simulink model "Proiect"  (R2023b)
settings: Solver=ode45  StartTime=0.0  StopTime=3600  RelTol=1e-3
values from neighbouring files (symbols this model uses):
  A = 332.5    [Proiect.m]
  C = 5.75    [Proiect.m]
  h = 12.99    [Proiect.m]
  h0 = 10.22    [Proiect.m]
  k = 0.025    [Proiect.m]
  k1 = 0.654    [Proiect.m]
  k11 = k2^2 + 4 * (k - k3) * k1    (= 0.0671946)    [Proiect.m]
  k12 = 8 * (k - k3)    (= 0.2048)    [Proiect.m]
  k13 = 2 * (k - k3)    (= 0.0512)    [Proiect.m]
  k2 = -0.015    [Proiect.m]
  k3 = -0.0006    [Proiect.m]
  k_compensare = kpFF/kp_comp    (= 0.13698630137)    [Proiect.m]
  k_eta = 8 * 10^(-5)    (= 8e-05)    [Proiect.m]
  ki2 = 0.184    [Proiect.m]
  kr = 2.1661    [Proiect.m]
  kr1 = Tf1/(kf1*T01)    (= 0.30303030303)    [Proiect.m]
  kr2 = Tf2/(kf2*T02)    (= 47.4368231047)    [Proiect.m]
  kre2 = 47.4    [Proiect.m]
  kri2 = 0.303    [Proiect.m]
  q = 32.45    [Proiect.m]
  q0 = 28.8    [Proiect.m]
  Ti = kr * 1/0.01589    (= 136.31843927)    [Proiect.m]
  Tr1 = Tf1    (= 0.76)    [Proiect.m]
  Tr2 = Tf2    (= 258.25)    [Proiect.m]
  u0 = 4.5    [Proiect.m]
libraries: slpidlib x12
(part 2 of 2)

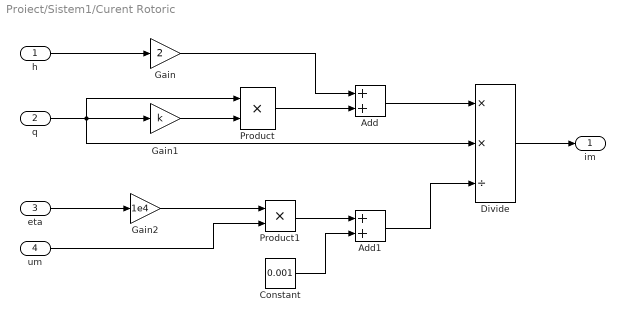
== system Proiect/Sistem1/Curent Rotoric ==
  h : Inport
  q : Inport  Port=2
  eta : Inport  Port=3
  um : Inport  Port=4
  Add : Sum
  Add1 : Sum
  Constant : Constant  Value=0.001
  Divide : Product  Inputs=**/
  Gain : Gain  Gain=2
  Gain1 : Gain  Gain=k
  Gain2 : Gain  Gain=1e4
  Product : Product
  Product1 : Product
  im : Outport
  wires:
  Gain1/1 -> Product/2
  Product/1 -> Add/2
  Gain2/1 -> Product1/1
  h/1 -> Gain/1
  Constant/1 -> Add1/2
  Gain/1 -> Add/1
  um/1 -> Product1/2
  Add1/1 -> Divide/3
  Divide/1 -> im/1
  Add/1 -> Divide/1
  q/1 -> Divide/2, Product/1, Gain1/1
  eta/1 -> Gain2/1
  Product1/1 -> Add1/1

== system Proiect/Sistem1/Filtru ==
  q : Inport
  Integrator : Integrator  InitialCondition=q0
  Sum : Sum  Inputs=|+-
  q_f : Outport
  wires:
  q/1 -> Sum/1
  Integrator/1 -> q_f/1, Sum/2
  Sum/1 -> Integrator/1

== system Proiect/Sistem1/Motor ==
  um : Inport
  im : Inport  Port=2
  Add : Sum  Inputs=+-
  Gain : Gain  Gain=3
  kn : Outport
  wires:
  im/1 -> Gain/1
  um/1 -> Add/1
  Add/1 -> kn/1
  Gain/1 -> Add/2

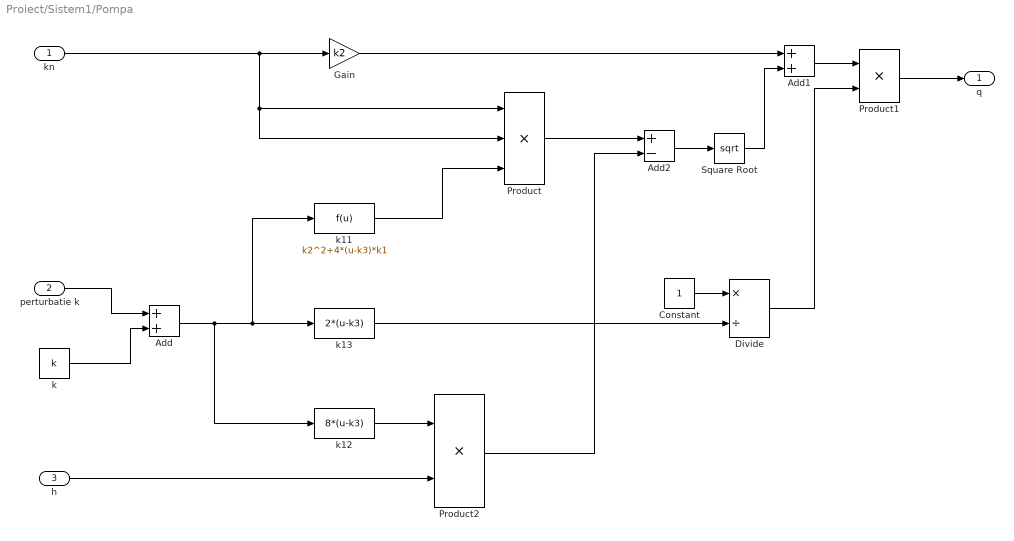
== system Proiect/Sistem1/Pompa ==
  kn : Inport
  perturbatie k : Inport  Port=2
  h : Inport  Port=3
  Add : Sum
  Add1 : Sum
  Add2 : Sum  Inputs=+-
  Constant : Constant
  Divide : Product  Inputs=*/
  Gain : Gain  Gain=k2
  Product : Product  Inputs=3
  Product1 : Product
  Product2 : Product
  Square Root : Sqrt
  k : Constant  Value=k
  k11 : Fcn  Expr=k2^2+4*(u-k3)*k1
  k12 : Fcn  Expr=8*(u-k3)
  k13 : Fcn  Expr=2*(u-k3)
  q : Outport
  wires:
  perturbatie k/1 -> Add/1
  k/1 -> Add/2
  k11/1 -> Product/3
  kn/1 -> Product/1, Product/2, Gain/1
  Gain/1 -> Add1/1
  Product/1 -> Add2/1
  Add2/1 -> Square Root/1
  Square Root/1 -> Add1/2
  Product1/1 -> q/1
  Add1/1 -> Product1/1
  Add/1 -> k12/1, k13/1, k11/1
  h/1 -> Product2/2
  Product2/1 -> Add2/2
  Constant/1 -> Divide/1
  k13/1 -> Divide/2
  Divide/1 -> Product1/2
  k12/1 -> Product2/1

== system Proiect/Sistem1/Randament Pompa ==
  q : Inport
  um : Inport  Port=2
  Gain : Gain  Gain=k_eta
  Product : Product
  eta : Outport
  wires:
  um/1 -> Gain/1
  Gain/1 -> Product/2
  Product/1 -> eta/1
  q/1 -> Product/1

== system Proiect/Sistem1/Rezervor ==
  q : Inport
  Fcn : Fcn  Expr=sqrt(u)*9
  Gain : Gain  Gain=1/A
  Integrator : Integrator  InitialCondition=h0
  Sum : Sum  Inputs=|+-
  h : Outport
  wires:
  Sum/1 -> Gain/1
  Integrator/1 -> Fcn/1, h/1
  q/1 -> Sum/1
  Gain/1 -> Integrator/1
  Fcn/1 -> Sum/2

== system Proiect/Sistem2/Amplificator ==
  ua : Inport
  Constant : Constant  Value=8.1
  Gain : Gain  Gain=2.2
  Gain1 : Gain  Gain=2.2
  Gain2 : Gain  Gain=5
  Saturation : Saturate  UpperLimit=22  LowerLimit=0
  Sum : Sum  Inputs=|++
  Sum1 : Sum  Inputs=|+-
  Switch : Switch  Threshold=8.1  SaturateOnIntegerOverflow=off  InputSameDT=off
  um : Outport
  wires:
  Switch/1 -> Saturation/1
  ua/1 -> Switch/2, Gain/1, Sum1/1, Gain1/1
  Gain1/1 -> Sum/1
  Gain2/1 -> Sum/2
  Saturation/1 -> um/1
  Gain/1 -> Switch/3
  Constant/1 -> Sum1/2
  Sum1/1 -> Gain2/1
  Sum/1 -> Switch/1

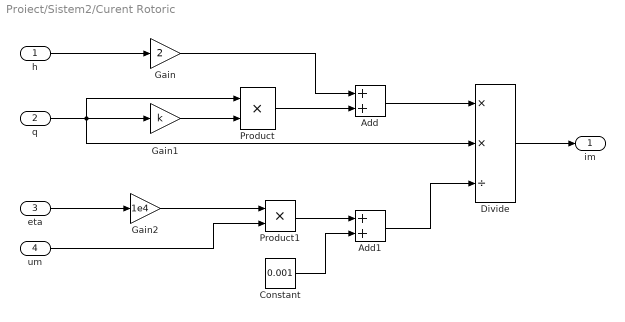
== system Proiect/Sistem2/Curent Rotoric ==
  h : Inport
  q : Inport  Port=2
  eta : Inport  Port=3
  um : Inport  Port=4
  Add : Sum
  Add1 : Sum
  Constant : Constant  Value=0.001
  Divide : Product  Inputs=**/
  Gain : Gain  Gain=2
  Gain1 : Gain  Gain=k
  Gain2 : Gain  Gain=1e4
  Product : Product
  Product1 : Product
  im : Outport
  wires:
  Gain1/1 -> Product/2
  Product/1 -> Add/2
  Gain2/1 -> Product1/1
  h/1 -> Gain/1
  Constant/1 -> Add1/2
  Gain/1 -> Add/1
  um/1 -> Product1/2
  Add1/1 -> Divide/3
  Divide/1 -> im/1
  Add/1 -> Divide/1
  q/1 -> Divide/2, Product/1, Gain1/1
  eta/1 -> Gain2/1
  Product1/1 -> Add1/1

== system Proiect/Sistem2/Filtru ==
  q : Inport
  Integrator : Integrator  InitialCondition=q0
  Sum : Sum  Inputs=|+-
  q_f : Outport
  wires:
  q/1 -> Sum/1
  Integrator/1 -> q_f/1, Sum/2
  Sum/1 -> Integrator/1

== system Proiect/Sistem2/Motor ==
  um : Inport
  im : Inport  Port=2
  Add : Sum  Inputs=+-
  Gain : Gain  Gain=3
  kn : Outport
  wires:
  im/1 -> Gain/1
  um/1 -> Add/1
  Add/1 -> kn/1
  Gain/1 -> Add/2

== system Proiect/Sistem2/Pompa ==
  kn : Inport
  h : Inport  Port=2
  Add : Sum
  Gain : Gain  Gain=k11
  Gain1 : Gain  Gain=k2
  Gain2 : Gain  Gain=1/k13
  Gain3 : Gain  Gain=k12
  Product : Product
  Square Root : Sqrt
  Subtract : Sum  Inputs=+-
  qi : Outport
  wires:
  Gain/1 -> Subtract/1
  Square Root/1 -> Add/2
  Gain3/1 -> Subtract/2
  Product/1 -> Gain/1
  Subtract/1 -> Square Root/1
  Gain2/1 -> qi/1
  kn/1 -> Product/1, Gain1/1, Product/2
  Add/1 -> Gain2/1
  Gain1/1 -> Add/1
  h/1 -> Gain3/1

== system Proiect/Sistem2/Randament Pompa ==
  q : Inport
  um : Inport  Port=2
  Gain : Gain  Gain=k_eta
  Product : Product
  eta : Outport
  wires:
  um/1 -> Gain/1
  Gain/1 -> Product/2
  Product/1 -> eta/1
  q/1 -> Product/1

== system Proiect/Sistem2/Rezervor ==
  q : Inport
  Add : Sum
  Constant : Constant  Value=C
  Gain : Gain  Gain=1/A
  Integrator : Integrator  InitialCondition=h0
  Product : Product
  Product1 : Product
  Square Root : Sqrt
  Step : Step  Time=500  After=2  SampleTime=0
  Sum : Sum  Inputs=|+-
  h : Outport
  perturbatie : Outport  Port=2
  qe : Outport  Port=3
  wires:
  Sum/1 -> Gain/1
  Integrator/1 -> Square Root/1, h/1
  q/1 -> Sum/1
  Gain/1 -> Integrator/1
  Product/1 -> qe/1, Sum/2
  Square Root/1 -> Product1/1, Product/1
  Add/1 -> Product/2
  Constant/1 -> Add/2
  Step/1 -> Product1/2, Add/1
  Product1/1 -> perturbatie/1

== system Proiect/Sistem3/Amplificator ==
  ua : Inport
  Constant : Constant  Value=8.1
  Gain : Gain  Gain=2.2
  Gain1 : Gain  Gain=2.2
  Gain2 : Gain  Gain=5
  Saturation : Saturate  UpperLimit=22  LowerLimit=0
  Sum : Sum  Inputs=|++
  Sum1 : Sum  Inputs=|+-
  Switch : Switch  Threshold=8.1  SaturateOnIntegerOverflow=off  InputSameDT=off
  um : Outport
  wires:
  Switch/1 -> Saturation/1
  ua/1 -> Switch/2, Gain/1, Sum1/1, Gain1/1
  Gain1/1 -> Sum/1
  Gain2/1 -> Sum/2
  Saturation/1 -> um/1
  Gain/1 -> Switch/3
  Constant/1 -> Sum1/2
  Sum1/1 -> Gain2/1
  Sum/1 -> Switch/1

== system Proiect/Sistem3/Curent Rotoric ==
  h : Inport
  q : Inport  Port=2
  eta : Inport  Port=3
  um : Inport  Port=4
  Add : Sum
  Add1 : Sum
  Constant : Constant  Value=0.001
  Divide : Product  Inputs=**/
  Gain : Gain  Gain=2
  Gain1 : Gain  Gain=k
  Gain2 : Gain  Gain=1e4
  Product : Product
  Product1 : Product
  im : Outport
  wires:
  Gain1/1 -> Product/2
  Product/1 -> Add/2
  Gain2/1 -> Product1/1
  h/1 -> Gain/1
  Constant/1 -> Add1/2
  Gain/1 -> Add/1
  um/1 -> Product1/2
  Add1/1 -> Divide/3
  Divide/1 -> im/1
  Add/1 -> Divide/1
  q/1 -> Divide/2, Product/1, Gain1/1
  eta/1 -> Gain2/1
  Product1/1 -> Add1/1

== system Proiect/Sistem3/Filtru ==
  q : Inport
  Integrator : Integrator  InitialCondition=q0
  Sum : Sum  Inputs=|+-
  q_f : Outport
  wires:
  q/1 -> Sum/1
  Integrator/1 -> q_f/1, Sum/2
  Sum/1 -> Integrator/1

== system Proiect/Sistem3/Motor ==
  um : Inport
  im : Inport  Port=2
  Add : Sum  Inputs=+-
  Gain : Gain  Gain=3
  kn : Outport
  wires:
  im/1 -> Gain/1
  um/1 -> Add/1
  Add/1 -> kn/1
  Gain/1 -> Add/2

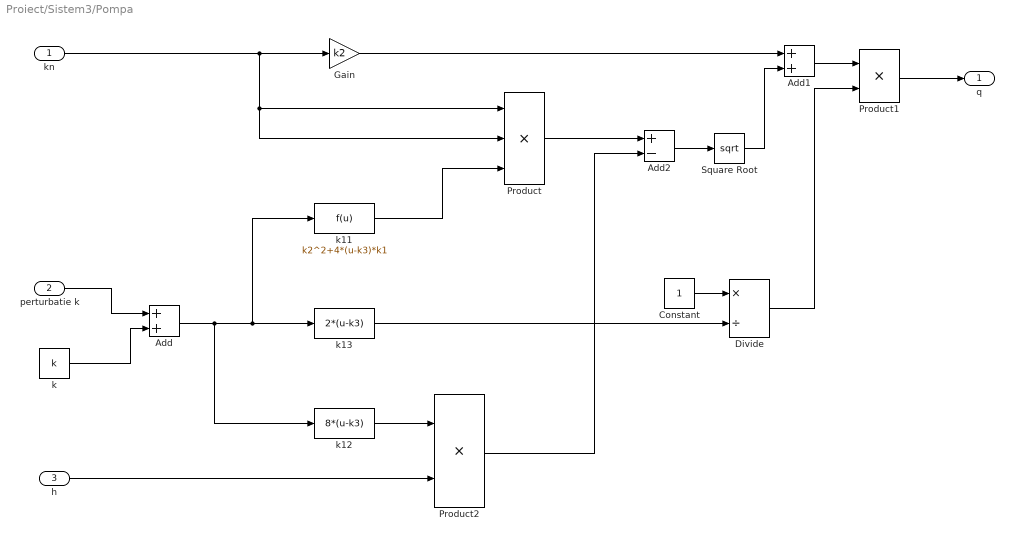
== system Proiect/Sistem3/Pompa ==
  kn : Inport
  perturbatie k : Inport  Port=2
  h : Inport  Port=3
  Add : Sum
  Add1 : Sum
  Add2 : Sum  Inputs=+-
  Constant : Constant
  Divide : Product  Inputs=*/
  Gain : Gain  Gain=k2
  Product : Product  Inputs=3
  Product1 : Product
  Product2 : Product
  Square Root : Sqrt
  k : Constant  Value=k
  k11 : Fcn  Expr=k2^2+4*(u-k3)*k1
  k12 : Fcn  Expr=8*(u-k3)
  k13 : Fcn  Expr=2*(u-k3)
  q : Outport
  wires:
  perturbatie k/1 -> Add/1
  k/1 -> Add/2
  k11/1 -> Product/3
  kn/1 -> Product/1, Product/2, Gain/1
  Gain/1 -> Add1/1
  Product/1 -> Add2/1
  Add2/1 -> Square Root/1
  Square Root/1 -> Add1/2
  Product1/1 -> q/1
  Add1/1 -> Product1/1
  Add/1 -> k12/1, k13/1, k11/1
  h/1 -> Product2/2
  Product2/1 -> Add2/2
  Constant/1 -> Divide/1
  k13/1 -> Divide/2
  Divide/1 -> Product1/2
  k12/1 -> Product2/1

== system Proiect/Sistem3/Randament Pompa ==
  q : Inport
  um : Inport  Port=2
  Gain : Gain  Gain=k_eta
  Product : Product
  eta : Outport
  wires:
  um/1 -> Gain/1
  Gain/1 -> Product/2
  Product/1 -> eta/1
  q/1 -> Product/1

== system Proiect/Sistem3/Rezervor ==
  q : Inport
  Fcn : Fcn  Expr=sqrt(u)*9
  Gain : Gain  Gain=1/A
  Integrator : Integrator  InitialCondition=h0
  Sum : Sum  Inputs=|+-
  h : Outport
  wires:
  Integrator/1 -> Fcn/1, h/1
  q/1 -> Sum/1
  Gain/1 -> Integrator/1
  Fcn/1 -> Sum/2
  Sum/1 -> Gain/1

== system Proiect/Sistem4/Amplificator ==
  ua : Inport
  Constant : Constant  Value=8.1
  Gain : Gain  Gain=2.2
  Gain1 : Gain  Gain=2.2
  Gain2 : Gain  Gain=5
  Saturation : Saturate  UpperLimit=22  LowerLimit=0
  Sum : Sum  Inputs=|++
  Sum1 : Sum  Inputs=|+-
  Switch : Switch  Threshold=8.1  SaturateOnIntegerOverflow=off  InputSameDT=off
  um : Outport
  wires:
  Switch/1 -> Saturation/1
  ua/1 -> Switch/2, Gain/1, Sum1/1, Gain1/1
  Gain1/1 -> Sum/1
  Gain2/1 -> Sum/2
  Saturation/1 -> um/1
  Gain/1 -> Switch/3
  Constant/1 -> Sum1/2
  Sum1/1 -> Gain2/1
  Sum/1 -> Switch/1

== system Proiect/Sistem4/Curent Rotoric ==
  h : Inport
  q : Inport  Port=2
  eta : Inport  Port=3
  um : Inport  Port=4
  Add : Sum
  Add1 : Sum
  Constant : Constant  Value=0.001
  Divide : Product  Inputs=**/
  Gain : Gain  Gain=2
  Gain1 : Gain  Gain=k
  Gain2 : Gain  Gain=1e4
  Product : Product
  Product1 : Product
  im : Outport
  wires:
  Gain1/1 -> Product/2
  Product/1 -> Add/2
  Gain2/1 -> Product1/1
  h/1 -> Gain/1
  Constant/1 -> Add1/2
  Gain/1 -> Add/1
  um/1 -> Product1/2
  Add1/1 -> Divide/3
  Divide/1 -> im/1
  Add/1 -> Divide/1
  q/1 -> Divide/2, Product/1, Gain1/1
  eta/1 -> Gain2/1
  Product1/1 -> Add1/1

== system Proiect/Sistem4/Filtru ==
  q : Inport
  Integrator : Integrator  InitialCondition=q0
  Sum : Sum  Inputs=|+-
  q_f : Outport
  wires:
  q/1 -> Sum/1
  Integrator/1 -> q_f/1, Sum/2
  Sum/1 -> Integrator/1

== system Proiect/Sistem4/Motor ==
  um : Inport
  im : Inport  Port=2
  Add : Sum  Inputs=+-
  Gain : Gain  Gain=3
  kn : Outport
  wires:
  im/1 -> Gain/1
  um/1 -> Add/1
  Add/1 -> kn/1
  Gain/1 -> Add/2

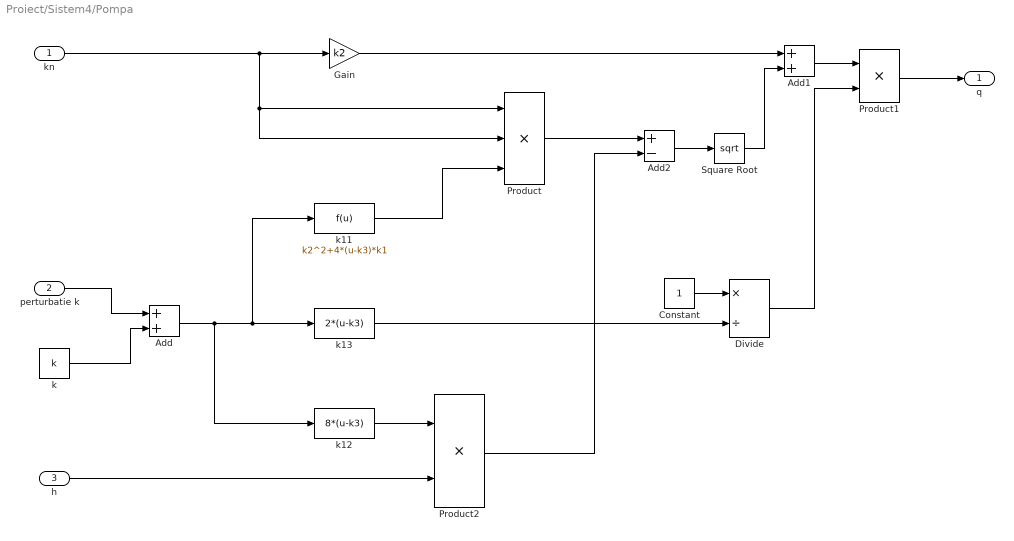
== system Proiect/Sistem4/Pompa ==
  kn : Inport
  perturbatie k : Inport  Port=2
  h : Inport  Port=3
  Add : Sum
  Add1 : Sum
  Add2 : Sum  Inputs=+-
  Constant : Constant
  Divide : Product  Inputs=*/
  Gain : Gain  Gain=k2
  Product : Product  Inputs=3
  Product1 : Product
  Product2 : Product
  Square Root : Sqrt
  k : Constant  Value=k
  k11 : Fcn  Expr=k2^2+4*(u-k3)*k1
  k12 : Fcn  Expr=8*(u-k3)
  k13 : Fcn  Expr=2*(u-k3)
  q : Outport
  wires:
  perturbatie k/1 -> Add/1
  k/1 -> Add/2
  k11/1 -> Product/3
  kn/1 -> Product/1, Product/2, Gain/1
  Gain/1 -> Add1/1
  Product/1 -> Add2/1
  Add2/1 -> Square Root/1
  Square Root/1 -> Add1/2
  Product1/1 -> q/1
  Add1/1 -> Product1/1
  Add/1 -> k12/1, k13/1, k11/1
  h/1 -> Product2/2
  Product2/1 -> Add2/2
  Constant/1 -> Divide/1
  k13/1 -> Divide/2
  Divide/1 -> Product1/2
  k12/1 -> Product2/1

== system Proiect/Sistem4/Randament Pompa ==
  q : Inport
  um : Inport  Port=2
  Gain : Gain  Gain=k_eta
  Product : Product
  eta : Outport
  wires:
  um/1 -> Gain/1
  Gain/1 -> Product/2
  Product/1 -> eta/1
  q/1 -> Product/1

== system Proiect/Sistem4/Rezervor ==
  q : Inport
  Fcn : Fcn  Expr=sqrt(u)*9
  Gain1 : Gain  Gain=1/A
  Integrator1 : Integrator  InitialCondition=h0
  Sum1 : Sum  Inputs=|+-
  h : Outport
  wires:
  Integrator1/1 -> Fcn/1, h/1
  q/1 -> Sum1/1
  Gain1/1 -> Integrator1/1
  Fcn/1 -> Sum1/2
  Sum1/1 -> Gain1/1

== system Proiect/Sistem5/Amplificator ==
  ua : Inport
  Constant : Constant  Value=8.1
  Gain : Gain  Gain=2.2
  Gain1 : Gain  Gain=2.2
  Gain2 : Gain  Gain=5
  Saturation : Saturate  UpperLimit=22  LowerLimit=0
  Sum : Sum  Inputs=|++
  Sum1 : Sum  Inputs=|+-
  Switch : Switch  Threshold=8.1  SaturateOnIntegerOverflow=off  InputSameDT=off
  um : Outport
  wires:
  Switch/1 -> Saturation/1
  ua/1 -> Switch/2, Gain/1, Sum1/1, Gain1/1
  Gain1/1 -> Sum/1
  Gain2/1 -> Sum/2
  Saturation/1 -> um/1
  Gain/1 -> Switch/3
  Constant/1 -> Sum1/2
  Sum1/1 -> Gain2/1
  Sum/1 -> Switch/1

== system Proiect/Sistem5/Curent Rotoric ==
  h : Inport
  q : Inport  Port=2
  eta : Inport  Port=3
  um : Inport  Port=4
  Add : Sum
  Add1 : Sum
  Constant : Constant  Value=0.001
  Divide : Product  Inputs=**/
  Gain : Gain  Gain=2
  Gain1 : Gain  Gain=k
  Gain2 : Gain  Gain=1e4
  Product : Product
  Product1 : Product
  im : Outport
  wires:
  Gain1/1 -> Product/2
  Product/1 -> Add/2
  Gain2/1 -> Product1/1
  h/1 -> Gain/1
  Constant/1 -> Add1/2
  Gain/1 -> Add/1
  um/1 -> Product1/2
  Add1/1 -> Divide/3
  Divide/1 -> im/1
  Add/1 -> Divide/1
  q/1 -> Divide/2, Product/1, Gain1/1
  eta/1 -> Gain2/1
  Product1/1 -> Add1/1

== system Proiect/Sistem5/Filtru ==
  q : Inport
  Integrator : Integrator  InitialCondition=q0
  Sum : Sum  Inputs=|+-
  q_f : Outport
  wires:
  q/1 -> Sum/1
  Integrator/1 -> q_f/1, Sum/2
  Sum/1 -> Integrator/1

== system Proiect/Sistem5/Motor ==
  um : Inport
  im : Inport  Port=2
  Add : Sum  Inputs=+-
  Gain : Gain  Gain=3
  kn : Outport
  wires:
  im/1 -> Gain/1
  um/1 -> Add/1
  Add/1 -> kn/1
  Gain/1 -> Add/2

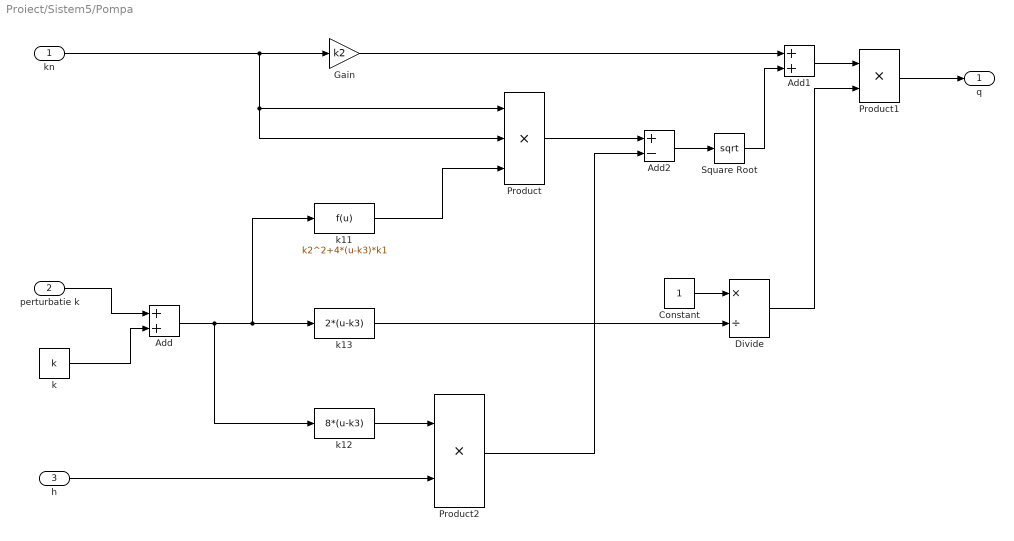
== system Proiect/Sistem5/Pompa ==
  kn : Inport
  perturbatie k : Inport  Port=2
  h : Inport  Port=3
  Add : Sum
  Add1 : Sum
  Add2 : Sum  Inputs=+-
  Constant : Constant
  Divide : Product  Inputs=*/
  Gain : Gain  Gain=k2
  Product : Product  Inputs=3
  Product1 : Product
  Product2 : Product
  Square Root : Sqrt
  k : Constant  Value=k
  k11 : Fcn  Expr=k2^2+4*(u-k3)*k1
  k12 : Fcn  Expr=8*(u-k3)
  k13 : Fcn  Expr=2*(u-k3)
  q : Outport
  wires:
  perturbatie k/1 -> Add/1
  k/1 -> Add/2
  k11/1 -> Product/3
  kn/1 -> Product/1, Product/2, Gain/1
  Gain/1 -> Add1/1
  Product/1 -> Add2/1
  Add2/1 -> Square Root/1
  Square Root/1 -> Add1/2
  Product1/1 -> q/1
  Add1/1 -> Product1/1
  Add/1 -> k12/1, k13/1, k11/1
  h/1 -> Product2/2
  Product2/1 -> Add2/2
  Constant/1 -> Divide/1
  k13/1 -> Divide/2
  Divide/1 -> Product1/2
  k12/1 -> Product2/1

== system Proiect/Sistem5/Randament Pompa ==
  q : Inport
  um : Inport  Port=2
  Gain : Gain  Gain=k_eta
  Product : Product
  eta : Outport
  wires:
  um/1 -> Gain/1
  Gain/1 -> Product/2
  Product/1 -> eta/1
  q/1 -> Product/1

== system Proiect/Sistem5/Rezervor ==
  q : Inport
  Add : Sum
  Constant : Constant  Value=C
  Gain : Gain  Gain=1/A
  Integrator : Integrator  InitialCondition=h0
  Product : Product
  Product1 : Product
  Square Root : Sqrt
  Step : Step  Time=250  After=2  SampleTime=0
  Sum : Sum  Inputs=|+-
  h : Outport
  perturbatie : Outport  Port=2
  wires:
  Product1/1 -> perturbatie/1
  Step/1 -> Product1/2, Add/1
  Constant/1 -> Add/2
  Square Root/1 -> Product1/1, Product/1
  Integrator/1 -> Square Root/1, h/1
  Add/1 -> Product/2
  Gain/1 -> Integrator/1
  Sum/1 -> Gain/1
  Product/1 -> Sum/2
  q/1 -> Sum/1

== system Proiect/Sistem6/Amplificator ==
  ua : Inport
  Constant : Constant  Value=8.1
  Gain : Gain  Gain=2.2
  Gain1 : Gain  Gain=2.2
  Gain2 : Gain  Gain=5
  Saturation : Saturate  UpperLimit=22  LowerLimit=0
  Sum : Sum  Inputs=|++
  Sum1 : Sum  Inputs=|+-
  Switch : Switch  Threshold=8.1  SaturateOnIntegerOverflow=off  InputSameDT=off
  um : Outport
  wires:
  Switch/1 -> Saturation/1
  ua/1 -> Switch/2, Gain/1, Sum1/1, Gain1/1
  Gain1/1 -> Sum/1
  Gain2/1 -> Sum/2
  Saturation/1 -> um/1
  Gain/1 -> Switch/3
  Constant/1 -> Sum1/2
  Sum1/1 -> Gain2/1
  Sum/1 -> Switch/1

== system Proiect/Sistem6/Curent Rotoric ==
  h : Inport
  q : Inport  Port=2
  eta : Inport  Port=3
  um : Inport  Port=4
  Add : Sum
  Add1 : Sum
  Constant : Constant  Value=0.001
  Divide : Product  Inputs=**/
  Gain : Gain  Gain=2
  Gain1 : Gain  Gain=k
  Gain2 : Gain  Gain=1e4
  Product : Product
  Product1 : Product
  im : Outport
  wires:
  Gain1/1 -> Product/2
  Product/1 -> Add/2
  Gain2/1 -> Product1/1
  h/1 -> Gain/1
  Constant/1 -> Add1/2
  Gain/1 -> Add/1
  um/1 -> Product1/2
  Add1/1 -> Divide/3
  Divide/1 -> im/1
  Add/1 -> Divide/1
  q/1 -> Divide/2, Product/1, Gain1/1
  eta/1 -> Gain2/1
  Product1/1 -> Add1/1

== system Proiect/Sistem6/Filtru ==
  q : Inport
  Integrator : Integrator  InitialCondition=q0
  Sum : Sum  Inputs=|+-
  q_f : Outport
  wires:
  q/1 -> Sum/1
  Integrator/1 -> q_f/1, Sum/2
  Sum/1 -> Integrator/1

== system Proiect/Sistem6/Motor ==
  um : Inport
  im : Inport  Port=2
  Add : Sum  Inputs=+-
  Gain : Gain  Gain=3
  kn : Outport
  wires:
  im/1 -> Gain/1
  um/1 -> Add/1
  Add/1 -> kn/1
  Gain/1 -> Add/2

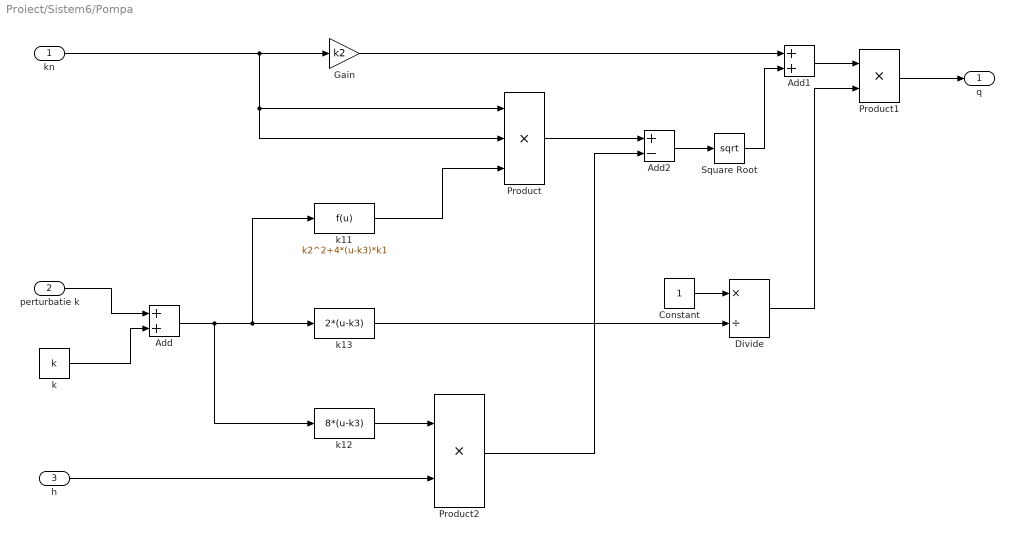
== system Proiect/Sistem6/Pompa ==
  kn : Inport
  perturbatie k : Inport  Port=2
  h : Inport  Port=3
  Add : Sum
  Add1 : Sum
  Add2 : Sum  Inputs=+-
  Constant : Constant
  Divide : Product  Inputs=*/
  Gain : Gain  Gain=k2
  Product : Product  Inputs=3
  Product1 : Product
  Product2 : Product
  Square Root : Sqrt
  k : Constant  Value=k
  k11 : Fcn  Expr=k2^2+4*(u-k3)*k1
  k12 : Fcn  Expr=8*(u-k3)
  k13 : Fcn  Expr=2*(u-k3)
  q : Outport
  wires:
  perturbatie k/1 -> Add/1
  k/1 -> Add/2
  k11/1 -> Product/3
  kn/1 -> Product/1, Product/2, Gain/1
  Gain/1 -> Add1/1
  Product/1 -> Add2/1
  Add2/1 -> Square Root/1
  Square Root/1 -> Add1/2
  Product1/1 -> q/1
  Add1/1 -> Product1/1
  Add/1 -> k12/1, k13/1, k11/1
  h/1 -> Product2/2
  Product2/1 -> Add2/2
  Constant/1 -> Divide/1
  k13/1 -> Divide/2
  Divide/1 -> Product1/2
  k12/1 -> Product2/1

== system Proiect/Sistem6/Randament Pompa ==
  q : Inport
  um : Inport  Port=2
  Gain : Gain  Gain=k_eta
  Product : Product
  eta : Outport
  wires:
  um/1 -> Gain/1
  Gain/1 -> Product/2
  Product/1 -> eta/1
  q/1 -> Product/1

== system Proiect/Sistem6/Rezervor ==
  q : Inport
  Fcn : Fcn  Expr=sqrt(u)*9
  Gain : Gain  Gain=1/A
  Integrator : Integrator  InitialCondition=h0
  Sum : Sum  Inputs=|+-
  h : Outport
  wires:
  Integrator/1 -> Fcn/1, h/1
  q/1 -> Sum/1
  Gain/1 -> Integrator/1
  Fcn/1 -> Sum/2
  Sum/1 -> Gain/1

== system Proiect/Sistem7/Amplificator ==
  ua : Inport
  Constant : Constant  Value=8.1
  Gain : Gain  Gain=2.2
  Gain1 : Gain  Gain=2.2
  Gain2 : Gain  Gain=5
  Saturation : Saturate  UpperLimit=22  LowerLimit=0
  Sum : Sum  Inputs=|++
  Sum1 : Sum  Inputs=|+-
  Switch : Switch  Threshold=8.1  SaturateOnIntegerOverflow=off  InputSameDT=off
  um : Outport
  wires:
  Switch/1 -> Saturation/1
  ua/1 -> Switch/2, Gain/1, Sum1/1, Gain1/1
  Gain1/1 -> Sum/1
  Gain2/1 -> Sum/2
  Saturation/1 -> um/1
  Gain/1 -> Switch/3
  Constant/1 -> Sum1/2
  Sum1/1 -> Gain2/1
  Sum/1 -> Switch/1

== system Proiect/Sistem7/Curent Rotoric ==
  h : Inport
  q : Inport  Port=2
  eta : Inport  Port=3
  um : Inport  Port=4
  Add : Sum
  Add1 : Sum
  Constant : Constant  Value=0.001
  Divide : Product  Inputs=**/
  Gain : Gain  Gain=2
  Gain1 : Gain  Gain=k
  Gain2 : Gain  Gain=1e4
  Product : Product
  Product1 : Product
  im : Outport
  wires:
  Gain1/1 -> Product/2
  Product/1 -> Add/2
  Gain2/1 -> Product1/1
  h/1 -> Gain/1
  Constant/1 -> Add1/2
  Gain/1 -> Add/1
  um/1 -> Product1/2
  Add1/1 -> Divide/3
  Divide/1 -> im/1
  Add/1 -> Divide/1
  q/1 -> Divide/2, Product/1, Gain1/1
  eta/1 -> Gain2/1
  Product1/1 -> Add1/1

== system Proiect/Sistem7/Filtru ==
  q : Inport
  Integrator : Integrator  InitialCondition=q0
  Sum : Sum  Inputs=|+-
  q_f : Outport
  wires:
  q/1 -> Sum/1
  Integrator/1 -> q_f/1, Sum/2
  Sum/1 -> Integrator/1

== system Proiect/Sistem7/Motor ==
  um : Inport
  im : Inport  Port=2
  Add : Sum  Inputs=+-
  Gain : Gain  Gain=3
  kn : Outport
  wires:
  im/1 -> Gain/1
  um/1 -> Add/1
  Add/1 -> kn/1
  Gain/1 -> Add/2

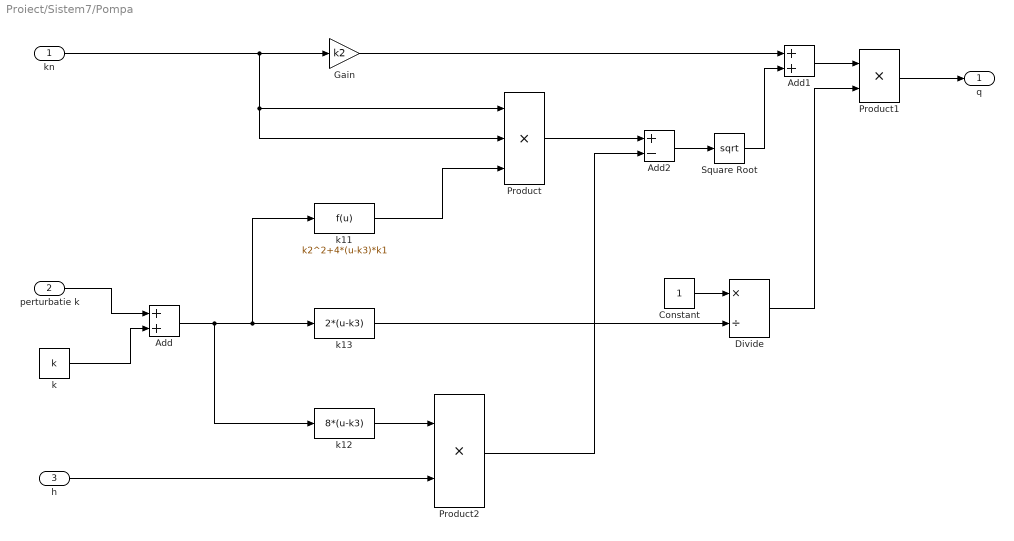
== system Proiect/Sistem7/Pompa ==
  kn : Inport
  perturbatie k : Inport  Port=2
  h : Inport  Port=3
  Add : Sum
  Add1 : Sum
  Add2 : Sum  Inputs=+-
  Constant : Constant
  Divide : Product  Inputs=*/
  Gain : Gain  Gain=k2
  Product : Product  Inputs=3
  Product1 : Product
  Product2 : Product
  Square Root : Sqrt
  k : Constant  Value=k
  k11 : Fcn  Expr=k2^2+4*(u-k3)*k1
  k12 : Fcn  Expr=8*(u-k3)
  k13 : Fcn  Expr=2*(u-k3)
  q : Outport
  wires:
  perturbatie k/1 -> Add/1
  k/1 -> Add/2
  k11/1 -> Product/3
  kn/1 -> Product/1, Product/2, Gain/1
  Gain/1 -> Add1/1
  Product/1 -> Add2/1
  Add2/1 -> Square Root/1
  Square Root/1 -> Add1/2
  Product1/1 -> q/1
  Add1/1 -> Product1/1
  Add/1 -> k12/1, k13/1, k11/1
  h/1 -> Product2/2
  Product2/1 -> Add2/2
  Constant/1 -> Divide/1
  k13/1 -> Divide/2
  Divide/1 -> Product1/2
  k12/1 -> Product2/1

== system Proiect/Sistem7/Randament Pompa ==
  q : Inport
  um : Inport  Port=2
  Gain : Gain  Gain=k_eta
  Product : Product
  eta : Outport
  wires:
  um/1 -> Gain/1
  Gain/1 -> Product/2
  Product/1 -> eta/1
  q/1 -> Product/1

== system Proiect/Sistem7/Rezervor ==
  q : Inport
  Fcn : Fcn  Expr=sqrt(u)*9
  Gain1 : Gain  Gain=1/A
  Integrator1 : Integrator  InitialCondition=h0
  Sum1 : Sum  Inputs=|+-
  h : Outport
  wires:
  Integrator1/1 -> Fcn/1, h/1
  q/1 -> Sum1/1
  Gain1/1 -> Integrator1/1
  Fcn/1 -> Sum1/2
  Sum1/1 -> Gain1/1
